simulink model "HostMotorControlClean"  (R2024a)
settings: Solver=FixedStepAuto  StartTime=0.0  StopTime=inf  FixedStep=Tscomms  RelTol=1e-3
values from neighbouring files (symbols this model uses):
  dataType = 'single'    [Para_Motor_Micro.m]
  Tscomms = 2*Ts*600    (= 0.036)    [Para_Motor_Micro.m]
libraries: instrumentseriallib x3
settings Model: Creator=axel_  LastModifiedBy=axel_
settings SolverCC: AlgebraicLoopSolver=TrustRegion
settings OptimizationCC: ReuseModelBlockBuffer=off
settings DebuggingCC: UnconnectedInputMsg=warning  UnconnectedOutputMsg=warning  UnconnectedLineMsg=warning
settings ModelReferenceCC: EnableRefExpFcnMdlSchedulingChecks=on
settings RTWCC: GPUComputeCapability=3.5  DLArmComputeVersion=19.05

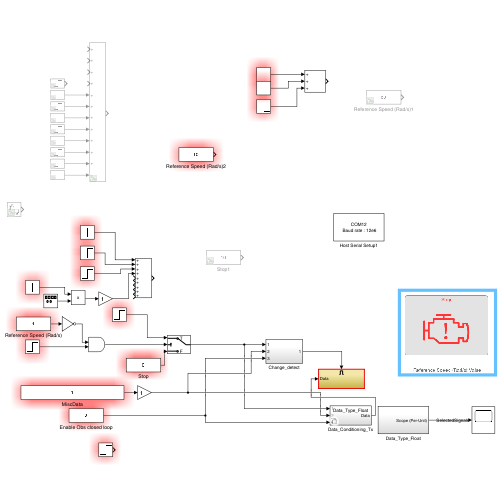
[thumbnail: Simulink's stored preview of the top-level diagram]
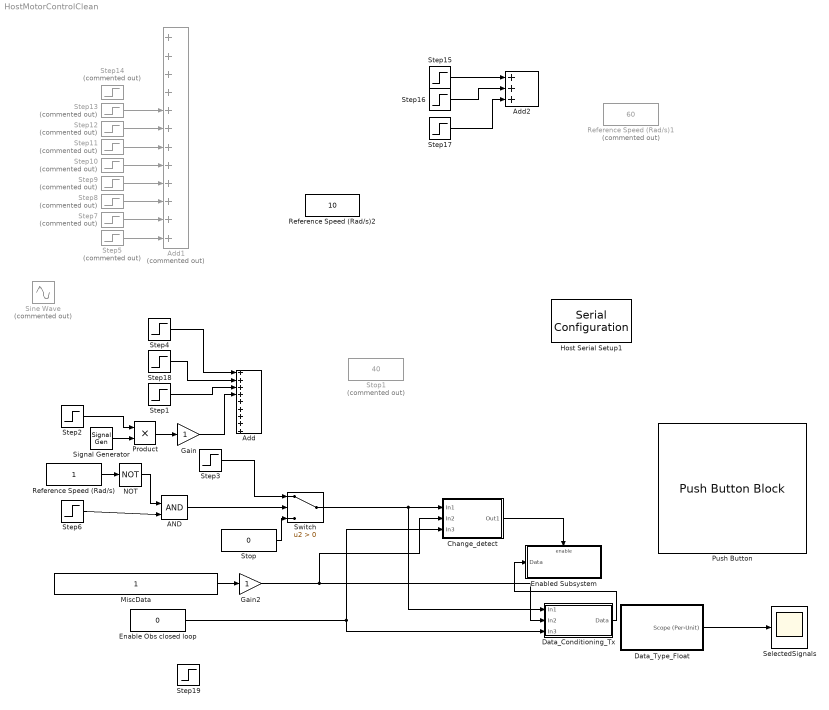
== system HostMotorControlClean ==
  AND : Logic  IconShape=distinctive  AllPortsSameDT=off  OutDataTypeStr=boolean
  Add : Sum  Inputs=+++++++++
  Add1 : Sum  Commented=on  Inputs=++++++++++++
  Add2 : Sum  Inputs=+++
  Change_detect : Subsystem
  Data_Conditioning_Tx : Subsystem  Variant=on
  Data_Type_Float : Subsystem  VariantControl=isequal(dataType, 'single')
  Enable Obs closed loop : Constant  Value=0  VectorParams1D=off  OutDataTypeStr=single  SampleTime=Tscomms
  Enabled Subsystem : Subsystem  TreatAsAtomicUnit=on
  Gain : Gain  OutDataTypeStr=single
  Gain2 : Gain  OutDataTypeStr=single
  Host Serial Setup1 : instrumentseriallib/Serial Configuration  Priority=-99  PortSel=COM12  Port=COM12  ComPort=COM12  BaudRate=12e6  DataBits=8  Parity=none  StopBits=1  ByteOrder=little-endian  FlowControl=none  Timeout=2  SimulateUsing=Interpreted execution  BlockInModel=on  aMode=5
  MiscData : Constant  VectorParams1D=off  OutDataTypeStr=single  SampleTime=Tscomms
  NOT : Logic  Operator=NOT  IconShape=distinctive  AllPortsSameDT=off  OutDataTypeStr=boolean
  Product : Product
  Push Button : PushButtonBlock  LabelPosition=Bottom  ButtonText=Stop  ButtonType=Latch  Icon=EngineFailure  IconAlignment=Bottom  IconColor=On  OffValue=0.000000
  Reference Speed (Rad/s) : Constant  VectorParams1D=off  OutDataTypeStr=single  SampleTime=Tscomms
  Reference Speed (Rad/s)1 : Constant  Commented=on  Value=60  VectorParams1D=off  OutDataTypeStr=single  SampleTime=Tscomms
  Reference Speed (Rad/s)2 : Constant  Value=10  VectorParams1D=off  OutDataTypeStr=single  SampleTime=Tscomms
  SelectedSignals : Scope
  Signal Generator : SignalGenerator  WaveForm=square  Amplitude=2  Frequency=0.5
  Sine Wave : Sin  Commented=on  Frequency=0.1  SampleTime=Tscomms
  Step1 : Step  Time=20  After=2.5  OutDataTypeStr=single  SampleTime=Tscomms
  Step10 : Step  Commented=on  Time=26  After=40  OutDataTypeStr=single  SampleTime=Tscomms
  Step11 : Step  Commented=on  Time=30  After=45  OutDataTypeStr=single  SampleTime=Tscomms
  Step12 : Step  Commented=on  Time=34  After=50  OutDataTypeStr=single  SampleTime=Tscomms
  Step13 : Step  Commented=on  Time=38  After=55  OutDataTypeStr=single  SampleTime=Tscomms
  Step14 : Step  Commented=on  Time=38  After=55  OutDataTypeStr=single  SampleTime=Tscomms
  Step15 : Step  Time=6  After=40  OutDataTypeStr=single  SampleTime=Tscomms
  Step16 : Step  Time=16  After=-30  OutDataTypeStr=single  SampleTime=Tscomms
  Step17 : Step  Time=18  After=-10  OutDataTypeStr=single  SampleTime=Tscomms
  Step18 : Step  Time=15  After=3  OutDataTypeStr=single  SampleTime=Tscomms
  Step19 : Step  Time=15  OutDataTypeStr=single  SampleTime=Tscomms
  Step2 : Step  Time=22  OutDataTypeStr=single  SampleTime=Tscomms
  Step3 : Step  Time=6  After=80  OutDataTypeStr=single  SampleTime=Tscomms
  Step4 : Step  Time=5  After=15  OutDataTypeStr=single  SampleTime=Tscomms
  Step5 : Step  Commented=on  Time=10  After=20  OutDataTypeStr=single  SampleTime=Tscomms
  Step6 : Step  Time=4  OutDataTypeStr=single  SampleTime=Tscomms
  Step7 : Step  Commented=on  Time=14  After=25  OutDataTypeStr=single  SampleTime=Tscomms
  Step8 : Step  Commented=on  Time=18  After=30  OutDataTypeStr=single  SampleTime=Tscomms
  Step9 : Step  Commented=on  Time=22  After=35  OutDataTypeStr=single  SampleTime=Tscomms
  Stop : Constant  Value=0  VectorParams1D=off  OutDataTypeStr=single  SampleTime=Tscomms
  Stop1 : Constant  Commented=on  Value=40  VectorParams1D=off  OutDataTypeStr=single  SampleTime=Tscomms
  Switch : Switch  Criteria=u2 > Threshold  SaturateOnIntegerOverflow=off  InputSameDT=off
  wires:
  Data_Conditioning_Tx/1(Data) -> Enabled Subsystem/1(Data)
  Enable Obs closed loop/1 -> Change_detect/3(In3), Data_Conditioning_Tx/3(In3)
  Change_detect/1(Out1) -> Enabled Subsystem/Enable
  Gain2/1 -> Change_detect/2(In2), Data_Conditioning_Tx/2(In2)
  AND/1 -> Switch/2
  Stop/1 -> Switch/3
  MiscData/1 -> Gain2/1
  NOT/1 -> AND/1
  Reference Speed (Rad/s)/1 -> NOT/1
  Step6/1 -> AND/2
  Step5/1 -> Add1/12
  Step7/1 -> Add1/11
  Step8/1 -> Add1/10
  Step9/1 -> Add1/9
  Step10/1 -> Add1/8
  Step11/1 -> Add1/7
  Step12/1 -> Add1/6
  Step13/1 -> Add1/5
  Data_Type_Float/1(Scope (Per-Unit)) -> SelectedSignals/1
  Step15/1 -> Add2/1
  Step16/1 -> Add2/2
  Step17/1 -> Add2/3
  Switch/1 -> Data_Conditioning_Tx/1(In1), Change_detect/1(In1)
  Step4/1 -> Add/1
  Step18/1 -> Add/2
  Step1/1 -> Add/3
  Signal Generator/1 -> Product/2
  Step2/1 -> Product/1
  Product/1 -> Gain/1
  Gain/1 -> Add/4
  Step3/1 -> Switch/1

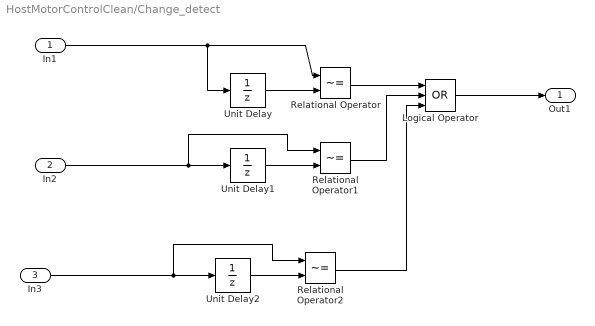
== system HostMotorControlClean/Change_detect ==
  In1 : Inport
  In2 : Inport  Port=2
  In3 : Inport  Port=3
  Logical Operator : Logic  Operator=OR  Inputs=3  AllPortsSameDT=off  OutDataTypeStr=boolean
  Relational Operator : RelationalOperator  Operator=~=  OutDataTypeStr=boolean  InputSameDT=off
  Relational Operator1 : RelationalOperator  Operator=~=  OutDataTypeStr=boolean  InputSameDT=off
  Relational Operator2 : RelationalOperator  Operator=~=  OutDataTypeStr=boolean  InputSameDT=off
  Unit Delay : UnitDelay  InitialCondition=0.5  SampleTime=-1  HasFrameUpgradeWarning=on
  Unit Delay1 : UnitDelay  SampleTime=-1  HasFrameUpgradeWarning=on
  Unit Delay2 : UnitDelay  SampleTime=-1  HasFrameUpgradeWarning=on
  Out1 : Outport  VectorParamsAs1DForOutWhenUnconnected=off
  wires:
  In2/1 -> Relational Operator1/1, Unit Delay1/1
  Relational Operator1/1 -> Logical Operator/2
  Unit Delay1/1 -> Relational Operator1/2
  Unit Delay/1 -> Relational Operator/2
  In1/1 -> Unit Delay/1, Relational Operator/1
  Relational Operator/1 -> Logical Operator/1
  Logical Operator/1 -> Out1/1
  Unit Delay2/1 -> Relational Operator2/2
  Relational Operator2/1 -> Logical Operator/3
  In3/1 -> Relational Operator2/1, Unit Delay2/1

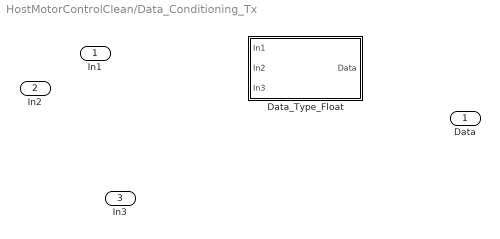
== system HostMotorControlClean/Data_Conditioning_Tx ==
  In1 : Inport
  In2 : Inport  Port=2
  In3 : Inport  Port=3
  Data_Type_Float : Subsystem  VariantControl=isequal(dataType, 'single')
  Data : Outport

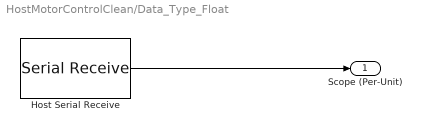
== system HostMotorControlClean/Data_Type_Float ==
  Host Serial Receive : instrumentseriallib/Serial Receive  PortSel=COM12  Port=COM12  ComPort=COM12  DataType=single  SaveDataType=uint8  ToggleHeader=on  Header='SSSS'  ToggleDataSize=on  DataSize=[600 2]  ToggleTerminator=on  Terminator=Custom terminator  CustomTerminator='EEEE'  InputFormat=Row major  EnableBlockingMode=on  ActionDataUnavailable=Output custom value  ActionWhenDataUnavailable=Output custom value  CustomValue=0.2  SampleTime=Tscomms  SimulateUsing=Interpreted execution  BlockInModel=on  aMode=5
      settings: LibrarySourceBlock=mcbhostblockslib/Host Serial Receive
  Scope (Per-Unit) : Outport
  wires:
  Host Serial Receive/1 -> Scope (Per-Unit)/1

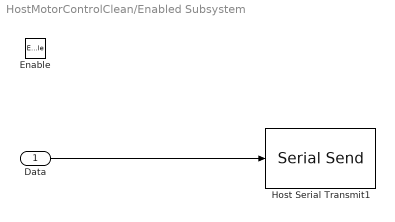
== system HostMotorControlClean/Enabled Subsystem ==
  Data : Inport
  Enable : EnablePort
  Host Serial Transmit1 : instrumentseriallib/Serial Send  PortSel=COM12  Port=COM12  ComPort=COM12  Header=[]  Terminator=<none>  CustomTerminator=[]  EnableBlockingMode=off  SimulateUsing=Interpreted execution  BlockInModel=on  aMode=5
  wires:
  Data/1 -> Host Serial Transmit1/1

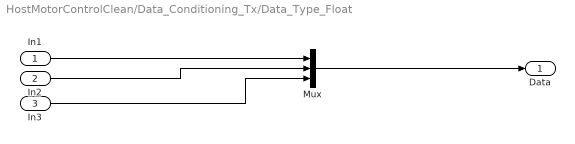
== system HostMotorControlClean/Data_Conditioning_Tx/Data_Type_Float ==
  In1 : Inport
  In2 : Inport  Port=2
  In3 : Inport  Port=3
  Mux : Mux  Inputs=3
  Data : Outport
  wires:
  In1/1 -> Mux/1
  Mux/1 -> Data/1
  In2/1 -> Mux/2
  In3/1 -> Mux/3
